simulink model "task2_lqr_lmi_modal"  (R2021b)
settings: Solver=FixedStepAuto  StartTime=0.0  StopTime=10  FixedStep=0.001  RelTol=1e-3
undefined symbols (not defined in the file): A, B, K3, K_lmi, K_modal, x0
settings Model: Creator=den  LastModifiedBy=den

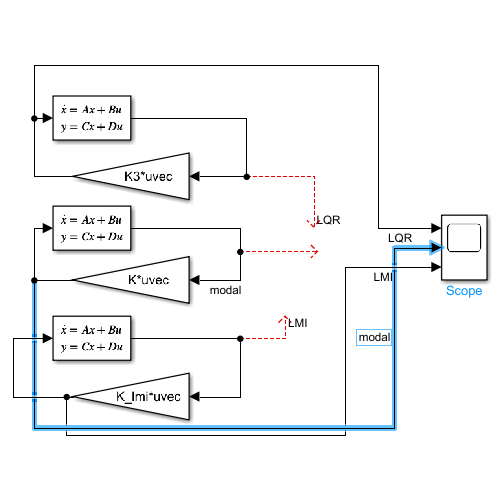
[thumbnail: Simulink's stored preview of the top-level diagram]
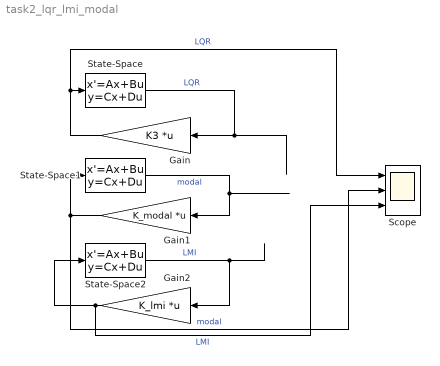
== system task2_lqr_lmi_modal ==
  Gain : Gain  Gain=K3  Multiplication=Matrix(K*u) (u vector)
  Gain1 : Gain  Gain=K_modal  Multiplication=Matrix(K*u) (u vector)
  Gain2 : Gain  Gain=K_lmi  Multiplication=Matrix(K*u) (u vector)
  Scope : Scope  NumInputPorts=3
  State-Space : StateSpace  A=A  B=B  C=[1 0 0 0; 0 1 0 0; 0 0 1 0; 0 0 0 1]  D=[ 0 0; 0 0; 0 0;0 0]  InitialCondition=x0
  State-Space1 : StateSpace  A=A  B=B  C=[1 0 0 0; 0 1 0 0; 0 0 1 0; 0 0 0 1]  D=[ 0 0; 0 0; 0 0;0 0]  InitialCondition=x0
  State-Space2 : StateSpace  A=A  B=B  C=[1 0 0 0; 0 1 0 0; 0 0 1 0; 0 0 0 1]  D=[ 0 0; 0 0; 0 0;0 0]  InitialCondition=x0
  wires:
  State-Space/1 -> Gain/1  "LQR"
  Gain/1 -> Scope/1, State-Space/1  "LQR"
  State-Space1/1 -> Gain1/1  "modal"
  Gain1/1 -> State-Space1/1, Scope/2  "modal"
  State-Space2/1 -> Gain2/1  "LMI"
  Gain2/1 -> Scope/3, State-Space2/1  "LMI"
